simulink model "LAB0_1"  (R2024b)
settings: Solver=ode45  StartTime=0.0  StopTime=.3  RelTol=1e-3
undefined symbols (not defined in the file or in its folder): Beq, daq, drv, gbox, Jeq, Kd_opt, Ki_opt, Kp_opt, mld, mot, rads2rpm, Req, sens, Tl
settings Model: Creator=Gioele  LastModifiedBy=Gioele
settings ConfigComp: CovBoundaryAbsTol=1.0e-5

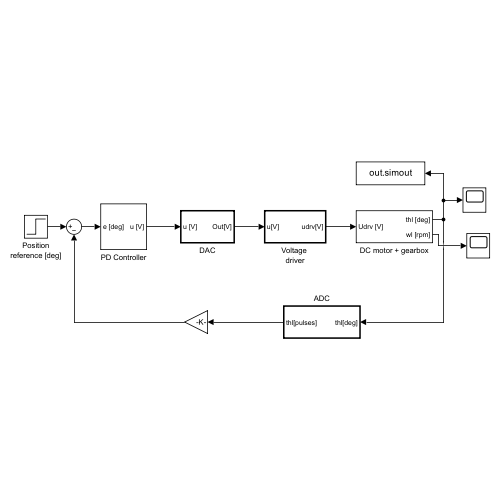
[thumbnail: Simulink's stored preview of the top-level diagram]
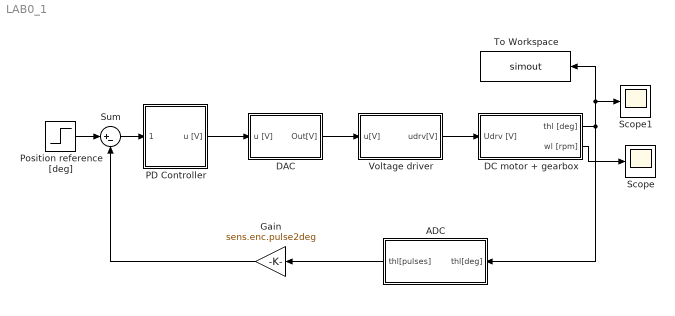
== system LAB0_1 ==
  ADC : Subsystem  TreatAsAtomicUnit=on
  DAC : Subsystem  TreatAsAtomicUnit=on
  DC motor + gearbox : Subsystem
  Gain : Gain  Gain=sens.enc.pulse2deg
  PD Controller : Subsystem
  Position reference [deg] : Step  Time=0  After=360  SampleTime=0
  Scope : Scope
  Scope1 : Scope
  Sum : Sum  Inputs=|+-
  To Workspace : ToWorkspace  VariableName=simout  SaveFormat=Timeseries  SampleTime=-1
  Voltage driver : Subsystem  TreatAsAtomicUnit=on
  wires:
  Voltage driver/1(udrv[V]) -> DC motor + gearbox/1(Udrv [V])
  DC motor + gearbox/2(wl [rpm]) -> Scope/1
  DAC/1(Out[V]) -> Voltage driver/1(u[V])
  ADC/1(thl[pulses]) -> Gain/1
  DC motor + gearbox/1(thl [deg]) -> ADC/1(thl[deg]), To Workspace/1, Scope1/1
  Position reference [deg]/1 -> Sum/1
  Sum/1 -> PD Controller/1(e [deg])
  Gain/1 -> Sum/2
  PD Controller/1(u [V]) -> DAC/1(u [V])

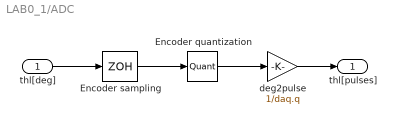
== system LAB0_1/ADC ==
  thl[deg] : Inport
  Encoder quantization : Quantizer  QuantizationInterval=daq.q
  Encoder sampling : ZeroOrderHold  SampleTime=daq.dac.Ts
  deg2pulse : Gain  Gain=1/daq.q
  thl[pulses] : Outport
  wires:
  Encoder quantization/1 -> deg2pulse/1
  thl[deg]/1 -> Encoder sampling/1
  Encoder sampling/1 -> Encoder quantization/1
  deg2pulse/1 -> thl[pulses]/1

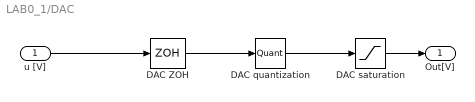
== system LAB0_1/DAC ==
  u [V] : Inport
  "DAC ZOH " : ZeroOrderHold  SampleTime=daq.dac.Ts
  DAC quantization : Quantizer  QuantizationInterval=daq.dac.q
  DAC saturation : Saturate  UpperLimit=daq.dac.fs  LowerLimit=-daq.dac.fs
  Out[V] : Outport
  wires:
  DAC quantization/1 -> DAC saturation/1
  u [V]/1 -> "DAC ZOH "/1
  "DAC ZOH "/1 -> DAC quantization/1
  DAC saturation/1 -> Out[V]/1

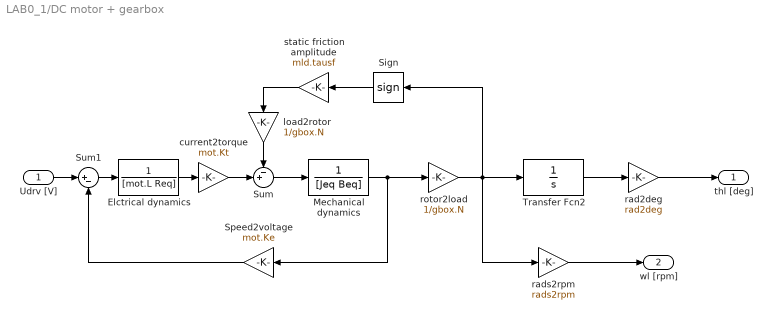
== system LAB0_1/DC motor + gearbox ==
  Udrv [V] : Inport
  Elctrical dynamics : TransferFcn  Denominator=[mot.L Req]
  Mechanical dynamics : TransferFcn  Denominator=[Jeq Beq]
  Sign : Signum  ZeroCross=off
  Speed2voltage : Gain  Gain=mot.Ke
  Sum : Sum  Inputs=-+|
  Sum1 : Sum  Inputs=|+-
  Transfer Fcn2 : TransferFcn  Denominator=[1 0]
  current2torque : Gain  Gain=mot.Kt
  load2rotor : Gain  Gain=1/gbox.N
  rad2deg : Gain  Gain=rad2deg
  rads2rpm : Gain  Gain=rads2rpm
  rotor2load : Gain  Gain=1/gbox.N
  static friction amplitude : Gain  Gain=mld.tausf
  thl [deg] : Outport
  wl [rpm] : Outport  Port=2
  wires:
  rotor2load/1 -> Sign/1, rads2rpm/1, Transfer Fcn2/1
  Sign/1 -> static friction amplitude/1
  rads2rpm/1 -> wl [rpm]/1
  Sum/1 -> Mechanical dynamics/1
  Udrv [V]/1 -> Sum1/1
  static friction amplitude/1 -> load2rotor/1
  load2rotor/1 -> Sum/1
  Transfer Fcn2/1 -> rad2deg/1
  current2torque/1 -> Sum/2
  Speed2voltage/1 -> Sum1/2
  Mechanical dynamics/1 -> Speed2voltage/1, rotor2load/1
  Elctrical dynamics/1 -> current2torque/1
  Sum1/1 -> Elctrical dynamics/1
  rad2deg/1 -> thl [deg]/1

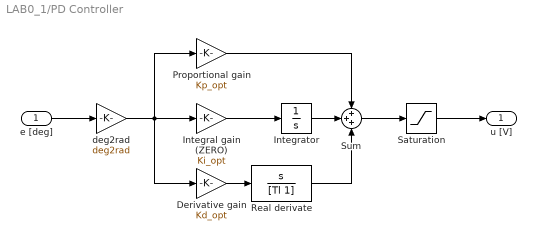
== system LAB0_1/PD Controller ==
  e [deg] : Inport
  Derivative gain : Gain  Gain=Kd_opt
  Integral gain (ZERO) : Gain  Gain=Ki_opt
  Integrator : Integrator
  Proportional gain : Gain  Gain=Kp_opt
  Real derivate : TransferFcn  Numerator=[1 0]  Denominator=[Tl 1]
  Saturation : Saturate  UpperLimit=daq.dac.fs  LowerLimit=-daq.dac.fs
  Sum : Sum  Inputs=+++
  deg2rad : Gain  Gain=deg2rad
  u [V] : Outport
  wires:
  Real derivate/1 -> Sum/3
  Integrator/1 -> Sum/2
  deg2rad/1 -> Proportional gain/1, Derivative gain/1, Integral gain (ZERO)/1
  Proportional gain/1 -> Sum/1
  e [deg]/1 -> deg2rad/1
  Derivative gain/1 -> Real derivate/1
  Sum/1 -> Saturation/1
  Saturation/1 -> u [V]/1
  Integral gain (ZERO)/1 -> Integrator/1

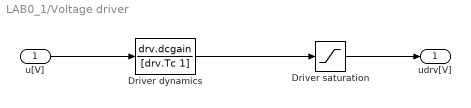
== system LAB0_1/Voltage driver ==
  u[V] : Inport
  Driver dynamics : TransferFcn  Numerator=drv.dcgain  Denominator=[drv.Tc 1]
  Driver saturation : Saturate  UpperLimit=drv.outmax  LowerLimit=-drv.outmax
  udrv[V] : Outport
  wires:
  Driver dynamics/1 -> Driver saturation/1
  u[V]/1 -> Driver dynamics/1
  Driver saturation/1 -> udrv[V]/1
